simulink model "traffic"  (R2021b)
settings: Solver=VariableStepAuto  StartTime=0.0  StopTime=10.0  RelTol=1e-3
settings Model: Creator=midol  LastModifiedBy=midol

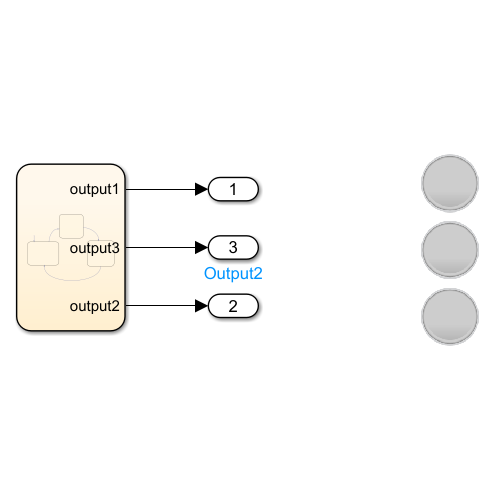
[thumbnail: Simulink's stored preview of the top-level diagram]
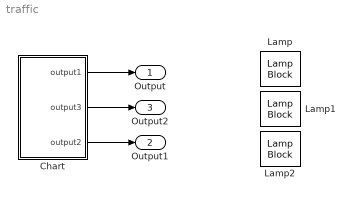
== system traffic ==
  Chart : Stateflow chart  TreatAsAtomicUnit=on
  Lamp : LampBlock  LabelPosition=Hide
  Lamp1 : LampBlock  LabelPosition=Hide
  Lamp2 : LampBlock  LabelPosition=Hide
  Output : Outport
  Output1 : Outport  Port=2
  Output2 : Outport  Port=3
  wires:
  Chart/1(output1) -> Output/1
  Chart/2(output3) -> Output2/1
  Chart/3(output2) -> Output1/1

== stateflow chart traffic/Chart ==
  state Yellow
    en:
    du:
    output2=1;
    ex:
    output2=0;
  state Red
    en:
    du:
    output3=1;
    ex:
    output3=0;
  state Green
    en:
    du:
    output1=1;
    ex:
    output1=0;
  Yellow -> Red : [after(10,tick)]
  Green -> Yellow : [after(10,tick)]
  (default) -> Green
  Red -> Green : [after(10,tick)]
  data: output1 output; output3 output; output2 output
